simulink model "ObstacleAvoidance"  (R2023a)
settings: Solver=ode4  StartTime=0.0  StopTime=T_stop  RelTol=1e-4  AbsTol=1e-4
StartFcn:
  | close all;
  | rho_cfrp = 6.32;
  | Ts = 1e-4;
  | Tsc = Ts;
undefined symbols (not defined in the file): k_air, Kii, Kiw, Kpi, Kpw, l_bat, miu_air, Opacity, p, planedepth, planex, planey, pr_air, T_stop, Temp, Vdc, X, xrot, Y, yrot, Z, zrot
libraries: sm_lib x356, nesl_utility x78, fl_lib x65, ee_lib x17, slpidlib x8, eeBldcCurrentController x4, eePwmGenerator x4, eeGeneralControl x4, test_library x4, batteryecm_lib x1
(part 1 of 8)
settings Model: Creator=tianwang  LastModifiedBy=ashih
settings SolverCC: AlgebraicLoopSolver=TrustRegion
settings OptimizationCC: DefaultParameterBehavior=Inlined  EnhancedBackFolding=on  PassReuseOutputArgsThreshold=0  OptimizeBlockOrder=speed  DifferentSizesBufferReuse=on  OptimizationCustomize=off
settings DebuggingCC: ParameterTunabilityLossMsg=error  UnconnectedInputMsg=warning  UnconnectedOutputMsg=warning  UnconnectedLineMsg=warning
settings ModelReferenceCC: EnableRefExpFcnMdlSchedulingChecks=on
settings SFSimCC: MATLABDynamicMemAlloc=off  CustomCodeUndefinedFunction=UseInterfaceOnly
settings RTWCC: GenerateReport=on  LaunchReport=on
settings CodeAppCC: ForceParamTrailComments=on  OperatorAnnotations=on
settings SimscapeCC: SimscapeLogType=all  SimscapeLogToSDI=on
settings DiagnosticsConfigSet: SimMechanicsRigidlyBoundBlock=none
settings ExplorerConfigSet: InternalSimMechanicsExplorerSettings="<ExplorerConfiguration><canonicalview>default</canonicalview><AnimationSetting><BasePlaybackSpeed>1.0</BasePlaybackSpeed><PlaybackSpeedFactor>1.0</PlaybackSpeedFactor></AnimationSetting><TilePanel><TileInfo><Tiles Columns=\"2\" Count=\"4\" Rows=\"2\"><Column Weight=\"0.5\"/><Column Weight=\"0.5\"/><Row Weight=\"0.4994\"/><Row Weight=\"0.5006\"/><Tile Height=\"1\" Width=\"1\" X=\"0\" Y=\"0\"/><Tile Height=\"1\" Width=\"1\" X=\"0\" Y=\"1\"/><Tile Height=\"1\" Width=\"1\" X=\"1\" Y=\"0\"/><Tile Height=\"1\" Width=\"1\" X=\"1\" Y=\"1\"/></Tiles></TileInfo><SceneInfo><SceneViewer><BGColor><R>0.60000002384185791</R><G>0.60000002384185791</G><B>0.60000002384185791</B></BGColor><Camera><DoPerspective>on</DoPerspective><Position><X>8.22328992273070902</X><Y>-3.04373425990231006</Y><Z>6.27152489428823401</Z></Position><Center><X>9.05691553848198261</X><Y>-7.3270363958746092</Y><Z>5.30243470030074171</Z></Center><Up><X>-0.0530873355813747533</X><Y>-0.230177435667943048</Y><Z>0.971699584702083063</Z></Up><ViewLimDist>1</ViewLimDist><YLim>0.466307658154998583</YLim><XLim>0.890324884305486508</XLim></Camera></SceneViewer><SceneViewer><BGColor><R>0.60000002384185791</R><G>0.60000002384185791</G><B>0.60000002384185791</B></BGColor><Camera><DoPerspective>off</DoPerspective><Position><X>5.00000000638571862</X><Y>-4.9999998855435237</Y><Z>12.4219790158057197</Z></Position><Center><X>5.00000000638571862</X><Y>-4.9999998855435237</Y><Z>2.97750008320821635</Z></Center><Up><X>0</X><Y>1</Y><Z>-0</Z></Up><ViewLimDist>1</ViewLimDist><YLim>5.66500000000000004</YLim><XLim>10.7904761904761894</XLim></Camera></SceneViewer><SceneViewer><BGColor><R>0.60000002384185791</R><G>0.60000002384185791</G><B>0.60000002384185791</B></BGColor><Camera><DoPerspective>off</DoPerspective><Position><X>-3.2794800033410807</X><Y>-5.06394715817210095</Y><Z>8.07533001389897898</Z></Position><Center><X>6.09563527499397484</X><Y>-5.35335986326467594</Y><Z>2.36240522021341448</Z></Center><Up><X>0.520298147861809168</X><Y>-0.00298968077239869512</Y><Z>0.853979448898186555</Z></Up><ViewLimDist>1</ViewLimDist><YLim>6.68440638643798035</YLim><XLim>12.762589759308792</XLim></Camera></SceneViewer><SceneViewer><BGColor><R>0.60000002384185791</R><G>0.60000002384185791</G><B>0.60000002384185791</B></BGColor><Camera><DoPerspective>off</DoPerspective><Position><X>11.1167954202289536</X><Y>-11.8295490480063652</Y><Z>6.79598621935422287</Z></Position><Center><X>5.09667302982083292</X><Y>-5.80942665759825161</Y><Z>0.775863828946114831</Z></Center><Up><X>-0.408248290463863073</X><Y>0.408248290463863073</Y><Z>0.816496580927726145</Z></Up><ViewLimDist>1</ViewLimDist><YLim>6.85015205426348484</YLim><XLim>13.047908674787589</XLim></Camera></SceneViewer></SceneInfo></TilePanel><MechEditorPanel><Cameras><Camera><Id>Camera1</Id><Value><Name>ride on the drone</Name><NativeCamera><PositionKeyframeSet><Keyframe><Time>0</Time><Value><X>-0.98102517823773216</X><Y>-5.4713411967234187</Y><Z>0.96761679727529326</Z></Value></Keyframe><Keyframe><Time>0.76000000000000001</Time><Value><X>-0.99261906360083585</X><Y>-5.5052148317158611</Y><Z>1.498055339667419</Z></Value></Keyframe><Keyframe><Time>1.74</Time><Value><X>-0.98102517823773216</X><Y>-5.555286722446434</Y><Z>3.1315459048019139</Z></Value></Keyframe><Keyframe><Time>2.5800000000000001</Time><Value><X>1.7790839250037722</X><Y>-5.5473623226265607</Y><Z>4.3656146773892459</Z></Value></Keyframe><Keyframe><Time>3.2800000000000002</Time><Value><X>2.7284590777804434</X><Y>-5.6139691649844634</Y><Z>5.2937584542701197</Z></Value></Keyframe><Keyframe><Time>5.6400000000000006</Time><Value><X>4.5026745101835584</X><Y>-5.6457503851239217</Y><Z>5.4148655689845642</Z></Value></Keyframe><Keyframe><Time>7.2960000000000003</Time><Value><X>7.6384098935542299</X><Y>-4.5525145479815734</Y><Z>8.3976329181318174</Z></Value></Keyframe><Keyframe><Time>11.92</Time><Value><X>7.6384098935542299</X><Y>-4.5525145479815734</Y><Z>8.3976329181318174</Z></Value></Keyframe><Keyframe><Time>13.108000000000001</Time><Value><X>8.223289922730709</X><Y>-3.0437342599023101</Y><Z>6.271524894288234</Z></Value></Keyframe></PositionKeyframeSet><CenterKeyframeSet><Keyframe><Time>0</Time><Value><X>7.5000000000000009</X><Y>-5.4713411967234187</Y><Z>0.96761679727529326</Z></Value></Keyframe><Keyframe><Time>0.76000000000000001</Time><Value><X>7.5000000045737156</X><Y>-5.5086734535529693</Y><Z>1.3291220515700248</Z></Value></Keyframe><Keyframe><Time>1.74</Time><Value><X>7.5000000000000009</X><Y>-5.555286722446434</Y><Z>3.1315459048019139</Z></Value></Keyframe><Keyframe><Time>2.5800000000000001</Time><Value><X>7.5</X><Y>-5.5473623226265607</Y><Z>4.3656146773892459</Z></Value></Keyframe><Keyframe><Time>3.2800000000000002</Time><Value><X>7.5</X><Y>-5.6139691649844634</Y><Z>5.2937584542701197</Z></Value></Keyframe><Keyframe><Time>5.6400000000000006</Time><Value><X>7.5</X><Y>-5.6457503851239217</Y><Z>5.4148655689845642</Z></Value></Keyframe><Keyframe><Time>7.2960000000000003</Time><Value><X>7.7294479865124739</X><Y>-4.754055561900703</Y><Z>6.0049999141429025</Z></Value></Keyframe><Keyframe><Time>11.92</Time><Value><X>7.7294479865124739</X><Y>-4.754055561900703</Y><Z>6.0049999141429016</Z></Value></Keyframe><Keyframe><Time>13.108000000000001</Time><Value><X>9.0569155384819826</X><Y>-7.3270363958746092</Y><Z>5.3024347003007417</Z></Value></Keyframe></CenterKeyframeSet><UpVectorKeyframeSet><Keyframe><Time>0</Time><Value><X>0</X><Y>0</Y><Z>1</Z></Value></Keyframe><Keyframe><Time>0.76000000000000001</Time><Value><X>0.019887839858441288</X><Y>-8.0993291557236055e-06</Y><Z>0.99980221732108898</Z></Value></Keyframe><Keyframe><Time>1.74</Time><Value><X>0</X><Y>0</Y><Z>1</Z></Value></Keyframe><Keyframe><Time>2.5800000000000001</Time><Value><X>0</X><Y>0</Y><Z>1</Z></Value></Keyframe><Keyframe><Time>3.2800000000000002</Time><Value><X>0</X><Y>0</Y><Z>1</Z></Value></Keyframe><Keyframe><Time>5.6400000000000006</Time><Value><X>0</X><Y>0</Y><Z>1</Z></Value></Keyframe><Keyframe><Time>7.2960000000000003</Time><Value><X>0.99863980522167117</X><Y>-0.032540807195370107</Y><Z>0.040738621649443037</Z></Value></Keyframe><Keyframe><Time>11.92</Time><Value><X>0.99863980522167128</X><Y>-0.0325408071953701</Y><Z>0.040738621649443113</Z></Value></Keyframe><Keyframe><Time>13.108000000000001</Time><Value><X>-0.053087335581374753</X><Y>-0.23017743566794305</Y><Z>0.97169958470208306</Z></Value></Keyframe></UpVectorKeyframeSet></NativeCamera></Value></Camera></Cameras><GfxPanelCameraMap><MapElement CameraMLId=\"Camera1\" GfxPanelIndex=\"0\"/></GfxPanelCameraMap><VideoCreator><PlaybackSpeedRatio>1.0</PlaybackSpeedRatio><FrameRate>60</FrameRate><VideoFormat>MPEG-4</VideoFormat><FrameSize>[1920 1080]</FrameSize></VideoCreator></MechEditorPanel></ExplorerConfiguration>"

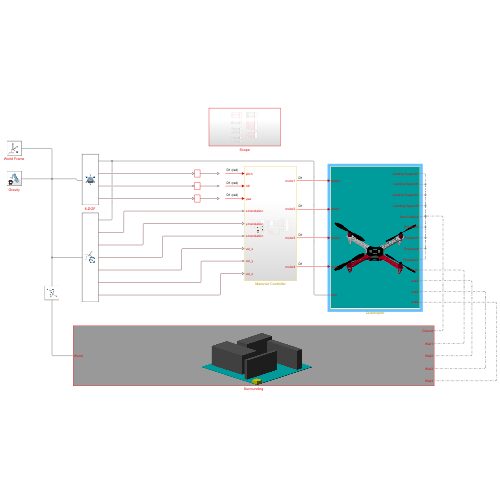
[thumbnail: Simulink's stored preview of the top-level diagram]
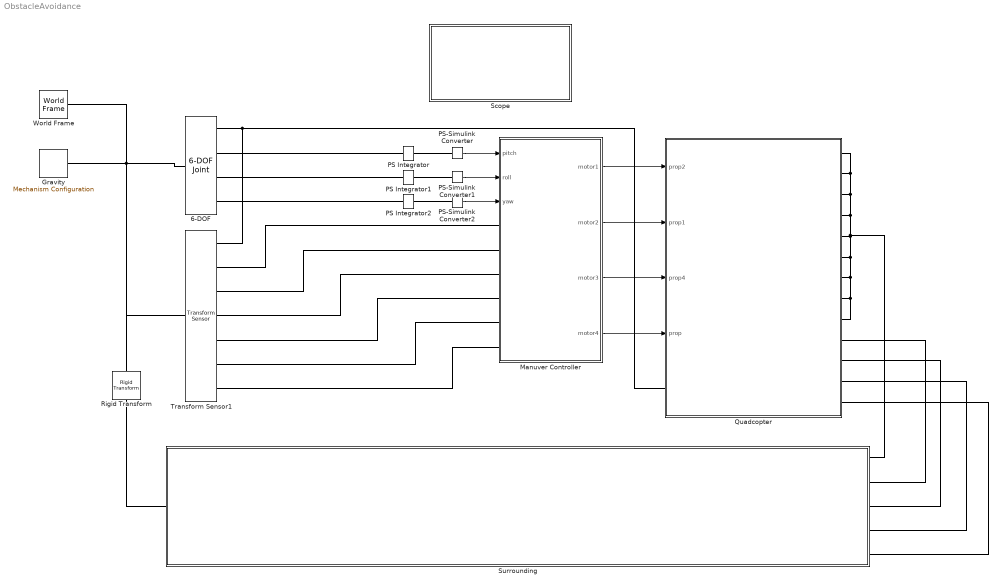
== system ObstacleAvoidance ==
  6-DOF : sm_lib/Joints/6-DOF Joint  JointMode=Normal  SenseConstraintForce=off  SenseConstraintForceX=off  SenseConstraintForceY=off  SenseConstraintForceZ=off  SenseConstraintTorque=off  SenseConstraintTorqueX=off  SenseConstraintTorqueY=off  SenseConstraintTorqueZ=off  SenseTotalForce=off  SenseTotalForceX=off  SenseTotalForceY=off  SenseTotalForceZ=off  SenseTotalTorque=off  SenseTotalTorqueX=off  SenseTotalTorqueY=off  SenseTotalTorqueZ=off  CompositeWrenchDir=FollowerOnBase  CompositeWrenchFrame=BaseFrame  PxEquilibriumPosition=0  PxEquilibriumPositionUnits=m  PxSpringStiffness=0  PxSpringStiffnessUnits=N/m  PxDampingCoefficient=0  PxDampingCoefficientUnits=N/(m/s)  PxTorqueActuationMode=NoTorque  PxMotionActuationMode=ComputedMotion  PxSensePosition=off  PxSenseVelocity=off  PxSenseAcceleration=off  PxSenseTorqueForce=off  PxSenseLowerLimitTorqueForce=off  PxSenseUpperLimitTorqueForce=off  PxLowerLimitSpecify=off  PxLowerLimitBound=-1  PxLowerLimitBoundUnits=m  PxLowerLimitStiffness=1e6  PxLowerLimitStiffnessUnits=N/m  PxLowerLimitDamping=1e3  PxLowerLimitDampingUnits=N/(m/s)  PxLowerLimitTransitionRegionWidth=1e-4  PxLowerLimitTransitionRegionWidthUnits=m  PxUpperLimitSpecify=off  PxUpperLimitBound=1  PxUpperLimitBoundUnits=m  PxUpperLimitStiffness=1e6  PxUpperLimitStiffnessUnits=N/m  PxUpperLimitDamping=1e3  PxUpperLimitDampingUnits=N/(m/s)  PxUpperLimitTransitionRegionWidth=1e-4  PxUpperLimitTransitionRegionWidthUnits=m  PxPositionTargetSpecify=on  PxPositionTargetPriority=High  PxPositionTargetValue=initial_x  PxPositionTargetValueUnits=m  PxVelocityTargetSpecify=off  PxVelocityTargetPriority=High  PxVelocityTargetValue=0  PxVelocityTargetValueUnits=m/s  PyEquilibriumPosition=0  PyEquilibriumPositionUnits=m  PySpringStiffness=0  PySpringStiffnessUnits=N/m  PyDampingCoefficient=0  PyDampingCoefficientUnits=N/(m/s)  PyTorqueActuationMode=NoTorque  PyMotionActuationMode=ComputedMotion  PySensePosition=off  PySenseVelocity=off  PySenseAcceleration=off  PySenseTorqueForce=off  PySenseLowerLimitTorqueForce=off  PySenseUpperLimitTorqueForce=off  PyLowerLimitSpecify=off  PyLowerLimitBound=-1  PyLowerLimitBoundUnits=m  PyLowerLimitStiffness=1e6  PyLowerLimitStiffnessUnits=N/m  PyLowerLimitDamping=1e3  PyLowerLimitDampingUnits=N/(m/s)  PyLowerLimitTransitionRegionWidth=1e-4  PyLowerLimitTransitionRegionWidthUnits=m  PyUpperLimitSpecify=off  PyUpperLimitBound=1  PyUpperLimitBoundUnits=m  PyUpperLimitStiffness=1e6  PyUpperLimitStiffnessUnits=N/m  PyUpperLimitDamping=1e3  PyUpperLimitDampingUnits=N/(m/s)  PyUpperLimitTransitionRegionWidth=1e-4  PyUpperLimitTransitionRegionWidthUnits=m  PyPositionTargetSpecify=on  PyPositionTargetPriority=High  PyPositionTargetValue=initial_y  PyPositionTargetValueUnits=m  PyVelocityTargetSpecify=off  PyVelocityTargetPriority=High  PyVelocityTargetValue=0  PyVelocityTargetValueUnits=m/s  PzEquilibriumPosition=0  PzEquilibriumPositionUnits=m  PzSpringStiffness=0  PzSpringStiffnessUnits=N/m  PzDampingCoefficient=0  PzDampingCoefficientUnits=N/(m/s)  PzTorqueActuationMode=NoTorque  PzMotionActuationMode=ComputedMotion  PzSensePosition=off  PzSenseVelocity=off  PzSenseAcceleration=off  PzSenseTorqueForce=off  PzSenseLowerLimitTorqueForce=off  PzSenseUpperLimitTorqueForce=off  PzLowerLimitSpecify=off  PzLowerLimitBound=-1  PzLowerLimitBoundUnits=m  PzLowerLimitStiffness=1e6  PzLowerLimitStiffnessUnits=N/m  PzLowerLimitDamping=1e3  PzLowerLimitDampingUnits=N/(m/s)  PzLowerLimitTransitionRegionWidth=1e-4  PzLowerLimitTransitionRegionWidthUnits=m  PzUpperLimitSpecify=off  PzUpperLimitBound=1  PzUpperLimitBoundUnits=m  PzUpperLimitStiffness=1e6  PzUpperLimitStiffnessUnits=N/m  PzUpperLimitDamping=1e3  PzUpperLimitDampingUnits=N/(m/s)  PzUpperLimitTransitionRegionWidth=1e-4  PzUpperLimitTransitionRegionWidthUnits=m  PzPositionTargetSpecify=on  PzPositionTargetPriority=High  PzPositionTargetValue=z0  PzPositionTargetValueUnits=m  PzVelocityTargetSpecify=off  PzVelocityTargetPriority=High  PzVelocityTargetValue=0  PzVelocityTargetValueUnits=m/s  SphEqPosRotationMethod=None  SphEqPosRotationAngleUnits=deg  SphEqPosRotationStandardAxis=+Z  SphEqPosRotationAngle=0.0  SphEqPosRotationArbitraryAxis=[0 0 1]  SphEqPosFollAlignAxisA=+X  SphEqPosBaseAlignAxisA=+Y  SphEqPosFollAlignAxisB=+Y  SphEqPosBaseAlignAxisB=+Z  SphEqPosRotationSequenceAxes=FollowerAxes  SphEqPosRotationSequence=XYX  SphEqPosRotationSequenceAngles=[0 0 0]  SphEqPosRotationSequenceAnglesUnits=deg  SphEqPosRotationMatrix=[1 0 0; 0 1 0; 0 0 1]  SphEqPosQuaternion=[1 0 0 0]  SphSpringStiffness=0  SphSpringStiffnessUnits=N*m/deg  SphDampingCoefficient=0  SphDampingCoefficientUnits=N*m/(deg/s)  SphActuateTorqueX=off  SphActuateTorqueY=off  SphActuateTorqueZ=off  SphActuateTorque=off  SphTorqueActuationMode=NoTorque  SphMotionActuationMode=ComputedMotion  SphActuationFrame=BaseFrame  SphSensePosition=off  SphSenseVelocityX=on  SphSenseVelocityY=on  SphSenseVelocityZ=on  SphSenseVelocity=off  SphSenseAccelerationX=off  SphSenseAccelerationY=off  SphSenseAccelerationZ=off  SphSenseAcceleration=off  SphSenseTorqueX=off  SphSenseTorqueY=off  SphSenseTorqueZ=off  SphSenseTorqueForce=off  SphSenseLowerLimitTorqueMag=off  SphSenseUpperLimitTorqueMag=off  SphSensingFrame=BaseFrame  SphLowerLimitSpecify=off  SphLowerLimitBound=15  SphLowerLimitBoundUnits=deg  SphLowerLimitStiffness=1e4  SphLowerLimitStiffnessUnits=N*m/deg  SphLowerLimitDamping=10  SphLowerLimitDampingUnits=N*m/(deg/s)  SphLowerLimitTransitionRegionWidth=0.1  SphLowerLimitTransitionRegionWidthUnits=deg  SphUpperLimitSpecify=off  SphUpperLimitBound=45  SphUpperLimitBoundUnits=deg  SphUpperLimitStiffness=1e4  SphUpperLimitStiffnessUnits=N*m/deg  SphUpperLimitDamping=10  SphUpperLimitDampingUnits=N*m/(deg/s)  SphUpperLimitTransitionRegionWidth=0.1  SphUpperLimitTransitionRegionWidthUnits=deg  SphPositionTargetRotationMethod=RotationSequence  SphPositionTargetRotationAngleUnits=deg  SphPositionTargetRotationStandardAxis=+Y  SphPositionTargetRotationAngle=0  SphPositionTargetRotationArbitraryAxis=[0 0 1]  SphPositionTargetFollAlignAxisA=+X  SphPositionTargetBaseAlignAxisA=+Y  SphPositionTargetFollAlignAxisB=+Y  SphPositionTargetBaseAlignAxisB=+Z  SphPositionTargetRotationSequenceAxes=FollowerAxes  SphPositionTargetRotationSequence=XYZ  SphPositionTargetRotationSequenceAngles=[xrot yrot zrot]  SphPositionTargetRotationSequenceAnglesUnits=deg  SphPositionTargetRotationMatrix=[1 0 0; 0 1 0; 0 0 1]  SphPositionTargetQuaternion=[1 0 0 0]  SphPositionTargetSpecify=on  SphPositionTargetPriority=High  SphVelocityTargetValue=[0 0 0]  SphVelocityTargetValueUnits=deg/s  SphVelocityTargetSpecify=off  SphVelocityTargetPriority=High  SphVelocityTargetInFollowerFrame=on
  Gravity : sm_lib/Utilities/Mechanism Configuration  UniformGravity=Constant  GravityVector=[0 0 -9.80665]  GravityVectorUnits=m/s^2  LinearizationDelta=0.001  JointModeTransitionNonlinearIterations=2
  Manuver Controller : Subsystem
  PS Integrator : fl_lib/Physical Signals/Linear Operators/PS Integrator  reset_method=foundation.enum.IntegratorResetSpec.None  initial_condition_spec=foundation.enum.IntegratorICSpec.Internal  saturation_spec=foundation.enum.IntegratorSaturationSpec.None  saturation_source_spec=foundation.enum.IntegratorSaturationSourceSpec.Internal  x0=0 rad  xu=inf s  xl=-inf s
  PS Integrator1 : fl_lib/Physical Signals/Linear Operators/PS Integrator  reset_method=foundation.enum.IntegratorResetSpec.None  initial_condition_spec=foundation.enum.IntegratorICSpec.Internal  saturation_spec=foundation.enum.IntegratorSaturationSpec.None  saturation_source_spec=foundation.enum.IntegratorSaturationSourceSpec.Internal  x0=0 rad  xu=inf s  xl=-inf s
  PS Integrator2 : fl_lib/Physical Signals/Linear Operators/PS Integrator  reset_method=foundation.enum.IntegratorResetSpec.None  initial_condition_spec=foundation.enum.IntegratorICSpec.Internal  saturation_spec=foundation.enum.IntegratorSaturationSpec.None  saturation_source_spec=foundation.enum.IntegratorSaturationSourceSpec.Internal  x0=0 rad  xu=inf s  xl=-inf s
  PS-Simulink Converter : nesl_utility/PS-Simulink Converter  PhysicalDomain=network_engine_domain  SubClassName=ps_output  LeftPortType=input  RightPortType=output  PseudoPeriodic=off  Frequencies=[]  VectorFormat=1-D array  Unit=inherit  AffineConversion=off
  PS-Simulink Converter1 : nesl_utility/PS-Simulink Converter  PhysicalDomain=network_engine_domain  SubClassName=ps_output  LeftPortType=input  RightPortType=output  PseudoPeriodic=off  Frequencies=[]  VectorFormat=1-D array  Unit=inherit  AffineConversion=off
  PS-Simulink Converter2 : nesl_utility/PS-Simulink Converter  PhysicalDomain=network_engine_domain  SubClassName=ps_output  LeftPortType=input  RightPortType=output  PseudoPeriodic=off  Frequencies=[]  VectorFormat=1-D array  Unit=inherit  AffineConversion=off
  Quadcopter : Subsystem
      mask Display: image('quad.PNG'); % Use "Edit Image" on toolstrip to change.
  Rigid Transform : sm_lib/Frames and Transforms/Rigid Transform  TranslationMethod=Cartesian  TranslationStandardOffset=0.05  TranslationStandardOffsetUnits=m  TranslationStandardAxis=-Z  TranslationCartesianOffset=[-5 5 -0.05]  TranslationCartesianOffsetUnits=m  TranslationROffset=0  TranslationROffsetUnits=m  TranslationZOffset=0  TranslationZOffsetUnits=m  TranslationThetaOffset=0  TranslationThetaOffsetUnits=deg  RotationMethod=None  RotationAngleUnits=deg  RotationStandardAxis=+Z  RotationAngle=0.0  RotationArbitraryAxis=[0 0 1]  FollAlignAxisA=+X  BaseAlignAxisA=+Y  FollAlignAxisB=+Y  BaseAlignAxisB=+Z  RotationSequenceAxes=FollowerAxes  RotationSequence=XYX  RotationSequenceAngles=[0 0 0]  RotationSequenceAnglesUnits=deg  RotationMatrix=[1 0 0; 0 1 0; 0 0 1]  Quaternion=[1 0 0 0]
  "Scope " : Subsystem
  Surrounding : Subsystem
      mask Display: image('surrounding.PNG'); % Use "Edit Image" on toolstrip to change.
  Transform Sensor1 : sm_lib/Frames and Transforms/Transform Sensor  MeasurementFrame=NonRotatingBase  RotationSequence=XYX  SenseAngle=off  SenseAxis=off  SenseQ=off  SenseR=off  SenseRotationSequence=off  SenseOmegaX=off  SenseOmegaY=off  SenseOmegaZ=off  SenseQDot=off  SenseRDot=off  SenseRotationSequenceDot=off  SenseAlphaX=off  SenseAlphaY=off  SenseAlphaZ=off  SenseQDDot=off  SenseRDDot=off  SenseX=on  SenseY=on  SenseZ=on  SenseRad=off  SenseAzim=off  SenseDist=off  SenseInc=off  SenseXDot=on  SenseYDot=on  SenseZDot=on  SenseRadDot=off  SenseAzimDot=off  SenseDistDot=off  SenseIncDot=off  SenseXDDot=off  SenseYDDot=off  SenseZDDot=off  SenseRadDDot=off  SenseAzimDDot=off  SenseDistDDot=off  SenseIncDDot=off
  World Frame : sm_lib/Frames and Transforms/World Frame
  wires:
  PS-Simulink Converter/1 -> Manuver Controller/1(pitch)
  PS-Simulink Converter1/1 -> Manuver Controller/2(roll)
  PS-Simulink Converter2/1 -> Manuver Controller/3(yaw)
  Manuver Controller/1(motor1) -> Quadcopter/1(prop2)
  Manuver Controller/2(motor2) -> Quadcopter/2("prop1 ")
  Manuver Controller/3(motor3) -> Quadcopter/3(prop4)
  Manuver Controller/4(motor4) -> Quadcopter/4(prop)
  connections:
  Quadcopter/LConn1 -- Transform Sensor1/RConn1 -- 6-DOF/RConn1
  Gravity/RConn1 -- Rigid Transform/RConn1 -- Transform Sensor1/LConn1 -- World Frame/RConn1 -- 6-DOF/LConn1
  Transform Sensor1/RConn2 -- Manuver Controller/LConn1
  PS Integrator/LConn1 -- 6-DOF/RConn2
  PS Integrator1/LConn1 -- 6-DOF/RConn3
  6-DOF/RConn4 -- PS Integrator2/LConn1
  PS-Simulink Converter2/LConn1 -- PS Integrator2/RConn1
  PS-Simulink Converter1/LConn1 -- PS Integrator1/RConn1
  PS-Simulink Converter/LConn1 -- PS Integrator/RConn1
  Transform Sensor1/RConn3 -- Manuver Controller/LConn2
  Transform Sensor1/RConn4 -- Manuver Controller/LConn3
  Transform Sensor1/RConn5 -- Manuver Controller/LConn4
  Transform Sensor1/RConn6 -- Manuver Controller/LConn5
  Transform Sensor1/RConn7 -- Manuver Controller/LConn6
  Quadcopter/RConn9 -- Quadcopter/RConn1 -- Quadcopter/RConn2 -- Quadcopter/RConn3 -- Quadcopter/RConn4 -- Surrounding/RConn1 -- Quadcopter/RConn5 -- Quadcopter/RConn6 -- Quadcopter/RConn7 -- Quadcopter/RConn8
  Surrounding/LConn1 -- Rigid Transform/LConn1
  Quadcopter/RConn10 -- Surrounding/RConn2
  Quadcopter/RConn11 -- Surrounding/RConn3
  Quadcopter/RConn12 -- Surrounding/RConn4
  Quadcopter/RConn13 -- Surrounding/RConn5

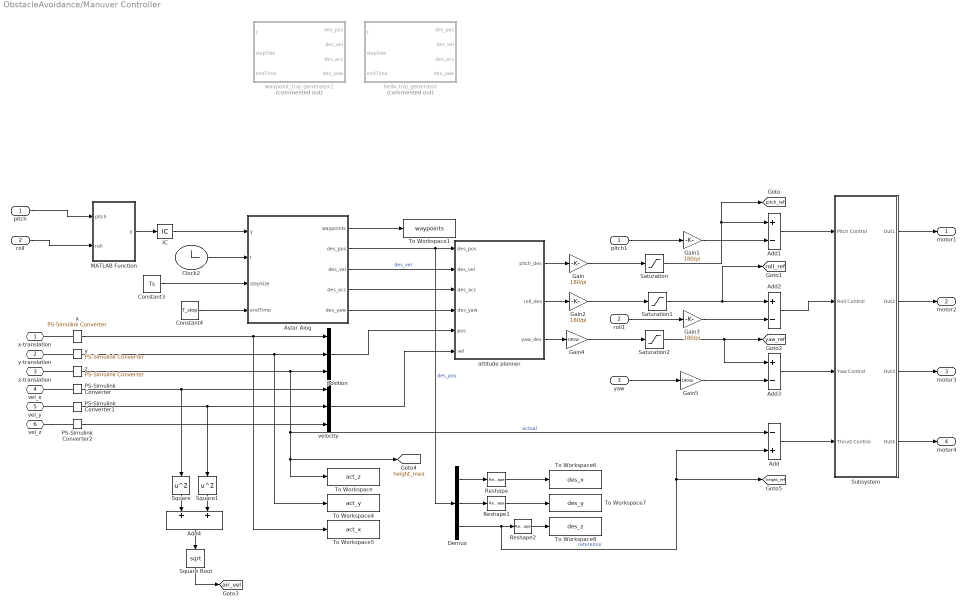
== system ObstacleAvoidance/Manuver Controller ==
  pitch : Inport
  roll : Inport  Port=2
  yaw : Inport  Port=3
  Add : Sum  Inputs=-+
  Add1 : Sum  Inputs=+-
  Add2 : Sum  Inputs=+-
  Add3 : Sum  Inputs=+-
  Add4 : Sum
  Astar Alog : MATLAB Function  TreatAsAtomicUnit=on
  Clock2 : Clock
  Constant3 : Constant  Value=Ts
  Constant4 : Constant  Value=T_stop
  Demux : Demux  Outputs=3
  Gain{,1..5} (6 alike) : Gain  Gain=180/pi
  IC : InitialCondition  Value=0
  MATLAB Function : MATLAB Function  TreatAsAtomicUnit=on
  PS-Simulink Converter : nesl_utility/PS-Simulink Converter  PhysicalDomain=network_engine_domain  SubClassName=ps_output  LeftPortType=input  RightPortType=output  PseudoPeriodic=off  Frequencies=[]  VectorFormat=1-D array  Unit=inherit  AffineConversion=off
  PS-Simulink Converter1 : nesl_utility/PS-Simulink Converter  PhysicalDomain=network_engine_domain  SubClassName=ps_output  LeftPortType=input  RightPortType=output  PseudoPeriodic=off  Frequencies=[]  VectorFormat=1-D array  Unit=inherit  AffineConversion=off
  PS-Simulink Converter2 : nesl_utility/PS-Simulink Converter  PhysicalDomain=network_engine_domain  SubClassName=ps_output  LeftPortType=input  RightPortType=output  PseudoPeriodic=off  Frequencies=[]  VectorFormat=1-D array  Unit=inherit  AffineConversion=off
  Reshape : Reshape
  Reshape1 : Reshape
  Reshape2 : Reshape
  Saturation : Saturate  UpperLimit=30  LowerLimit=-30
  Saturation1 : Saturate  UpperLimit=30  LowerLimit=-30
  Saturation2 : Saturate  UpperLimit=30  LowerLimit=-30
  Square : Math  Operator=square
  Square Root : Sqrt
  Square1 : Math  Operator=square
  Subsystem : Subsystem
  To Workspace : ToWorkspace  VariableName=act_z  SampleTime=-1
  To Workspace1 : ToWorkspace  VariableName=waypoints  SampleTime=-1
  To Workspace4 : ToWorkspace  VariableName=act_y  SampleTime=-1
  To Workspace5 : ToWorkspace  VariableName=act_x  SampleTime=-1
  To Workspace6 : ToWorkspace  VariableName=des_x  SampleTime=-1
  To Workspace7 : ToWorkspace  VariableName=des_y  SampleTime=-1
  To Workspace8 : ToWorkspace  VariableName=des_z  SampleTime=-1
  attitude planner : MATLAB Function  TreatAsAtomicUnit=on
  helix_traj_generator : MATLAB Function  Commented=on  TreatAsAtomicUnit=on
  pitch1 : InportShadow
  position : Mux  Inputs=3
  roll1 : InportShadow  Port=2
  velocity : Mux  Inputs=3
  waypoint_traj_generator2 : MATLAB Function  Commented=on  TreatAsAtomicUnit=on
  x : nesl_utility/PS-Simulink Converter  PhysicalDomain=network_engine_domain  SubClassName=ps_output  LeftPortType=input  RightPortType=output  PseudoPeriodic=off  Frequencies=[]  VectorFormat=1-D array  Unit=1  AffineConversion=off
  y : nesl_utility/PS-Simulink Converter  PhysicalDomain=network_engine_domain  SubClassName=ps_output  LeftPortType=input  RightPortType=output  PseudoPeriodic=off  Frequencies=[]  VectorFormat=1-D array  Unit=1  AffineConversion=off
  z : nesl_utility/PS-Simulink Converter  PhysicalDomain=network_engine_domain  SubClassName=ps_output  LeftPortType=input  RightPortType=output  PseudoPeriodic=off  Frequencies=[]  VectorFormat=1-D array  Unit=1  AffineConversion=off
  x-translation : PMIOPort  Side=Left
  y-translation : PMIOPort  Port=2  Side=Left
  z-translation : PMIOPort  Port=3  Side=Left
  vel_x : PMIOPort  Port=4  Side=Left
  vel_y : PMIOPort  Port=5  Side=Left
  vel_z : PMIOPort  Port=6  Side=Left
  motor1 : Outport
  motor2 : Outport  Port=2
  motor3 : Outport  Port=3
  motor4 : Outport  Port=4
  tag scope: air_vel=global, height_mea=global, height_ref=global, pitch_ref=global, roll_ref=global, yaw_ref=global
  wires:
  Subsystem/1(Out1) -> motor1/1
  Add1/1 -> Subsystem/1(Pitch Control)
  Add3/1 -> Subsystem/3(Yaw Control)
  attitude planner/3(yaw_des) -> Gain4/1
  velocity/1 -> attitude planner/6(vel)
  z/1 -> [height_mea], To Workspace/1, Add/1, position/3  "actual"
  PS-Simulink Converter1/1 -> Square1/1, velocity/2
  PS-Simulink Converter/1 -> Square/1, velocity/1
  PS-Simulink Converter2/1 -> velocity/3
  Gain5/1 -> Add3/2
  x/1 -> To Workspace5/1, position/1
  Gain2/1 -> Saturation1/1
  Gain4/1 -> Saturation2/1
  Add/1 -> Subsystem/4(Thrust Control)
  Subsystem/2(Out2) -> motor2/1
  Gain/1 -> Saturation/1
  Subsystem/4(Out4) -> motor4/1
  Astar Alog/5(des_yaw) -> attitude planner/4(des_yaw)
  attitude planner/2(roll_des) -> Gain2/1
  Add2/1 -> Subsystem/2(Roll Control)
  position/1 -> attitude planner/5(pos)
  attitude planner/1(pitch_des) -> Gain/1
  Astar Alog/4(des_acc) -> attitude planner/3(des_acc)
  Demux/2 -> Reshape1/1
  Demux/1 -> Reshape/1
  Astar Alog/3(des_vel) -> attitude planner/2(des_vel)  "des_vel"
  Demux/3 -> [height_ref], Add/2, Reshape2/1  "reference"
  Subsystem/3(Out3) -> motor3/1
  Astar Alog/2(des_pos) -> Demux/1, attitude planner/1(des_pos)  "des_pos"
  y/1 -> To Workspace4/1, position/2
  Constant4/1 -> Astar Alog/4(endTime)
  Constant3/1 -> Astar Alog/3(stepSize)
  Clock2/1 -> Astar Alog/2(t)
  Gain1/1 -> Add1/2
  Gain3/1 -> Add2/2
  Astar Alog/1(waypoints) -> To Workspace1/1
  Square/1 -> Add4/1
  Square1/1 -> Add4/2
  Add4/1 -> Square Root/1
  Square Root/1 -> [air_vel]
  Saturation/1 -> Add1/1, [pitch_ref]
  Saturation1/1 -> [roll_ref], Add2/1
  Saturation2/1 -> [yaw_ref], Add3/1
  MATLAB Function/1(y) -> IC/1
  pitch/1 -> MATLAB Function/1(pitch)
  roll/1 -> MATLAB Function/2(roll)
  roll1/1 -> Gain3/1
  pitch1/1 -> Gain1/1
  IC/1 -> Astar Alog/1(y)
  yaw/1 -> Gain5/1
  Reshape/1 -> To Workspace6/1
  Reshape1/1 -> To Workspace7/1
  Reshape2/1 -> To Workspace8/1
  connections:
  y/LConn1 -- y-translation/RConn1
  x/LConn1 -- x-translation/RConn1
  PS-Simulink Converter/LConn1 -- vel_x/RConn1
  z/LConn1 -- z-translation/RConn1
  PS-Simulink Converter1/LConn1 -- vel_y/RConn1
  vel_z/RConn1 -- PS-Simulink Converter2/LConn1

== system ObstacleAvoidance/Quadcopter ==
  prop2 : Inport
  "prop1 " : Inport  Port=2
  prop4 : Inport  Port=3
  prop : Inport  Port=4
  PS-Simulink Converter{,1..3} (4 alike) : nesl_utility/PS-Simulink Converter  PhysicalDomain=network_engine_domain  SubClassName=ps_output  LeftPortType=input  RightPortType=output  PseudoPeriodic=off  Frequencies=[]  VectorFormat=1-D array  Unit=inherit  AffineConversion=off
  Spatial Contact Force{,1..3} (4 alike) : sm_lib/Forces and Torques/Spatial Contact Force  SenseContactBaseRotation=off  SenseContactBaseTranslation=off  CoefficientOfDynamicFriction=0.1  CoefficientOfStaticFriction=0.25  NormalDamping=1e3  NormalDampingUnits=N/(m/s)  SenseContactSignal=off  NormalStiffness=1e6  NormalStiffnessUnits=N/m  FrictionalCriticalVelocity=1e-3  FrictionalCriticalVelocityUnits=m/s  ZeroCrossDetectContactStartAndEnd=off  SenseContactFollowerRotation=off  SenseContactFollowerTranslation=off  FrictionType=SmoothStickSlip  SenseFrictionalForceMagnitude=off  SenseNormalForceMagnitude=off  NormalForceType=SmoothSpringDamper  SenseNormalVelocity=off  SenseSeparationDistance=off  SenseTangentialVelocity=off  NormalTransitionRegionWidth=1e-4  NormalTransitionRegionWidthUnits=m
  battery : Subsystem
  propeller1 : Subsystem
      mask Display: image('prop2.PNG'); % Use "Edit Image" on toolstrip to change.
  propeller2 : Subsystem
      mask Display: image('prop1.PNG'); % Use "Edit Image" on toolstrip to change.
  "propeller3 " : Subsystem
      mask Display: image('prop4.PNG'); % Use "Edit Image" on toolstrip to change.
  propeller4 : Subsystem
      mask Display: image('prop3.PNG'); % Use "Edit Image" on toolstrip to change.
  quad_body : Subsystem  mask{GraphicOpacity=Opacity}
      mask prompts: GraphicOpacity "Detector Opacity:"
      mask TypeOptions GraphicOpacity: Spherical Solid/GraphicOpacity | Spherical Solid1/GraphicOpacity | Spherical Solid2/GraphicOpacity | Spherical Solid3/GraphicOpacity
      mask DialogControl DescGroupVar Prompt: QuadcopterBodyCollisionSetup
      mask DialogControl DescTextVar Prompt: The subsystem sets up the collision between the propeller, ground and wall.
      mask Display: image('quad_body.PNG'); % Use "Edit Image" on toolstrip to change.
  "Landing Support2 " : PMIOPort  Side=Right
  Landing Support1 : PMIOPort  Port=2  Side=Right
  arm : PMIOPort  Port=3  Side=Left
  "Landing Support4 " : PMIOPort  Port=4  Side=Right
  Landing Support3 : PMIOPort  Port=5  Side=Right
  Arm Collision : PMIOPort  Port=6  Side=Right
  Propeller2 : PMIOPort  Port=7  Side=Right
  Propeller1 : PMIOPort  Port=8  Side=Right
  Propeller4 : PMIOPort  Port=9  Side=Right
  "Propeller3 " : PMIOPort  Port=10  Side=Right
  wall1 : PMIOPort  Port=11  Side=Right
  wall2 : PMIOPort  Port=12  Side=Right
  wall3 : PMIOPort  Port=13  Side=Right
  wall4 : PMIOPort  Port=14  Side=Right
  tag scope: T1=global, T2=global, T3=global, T4=global
  wires:
  PS-Simulink Converter/1 -> [T2]
  PS-Simulink Converter1/1 -> [T4]
  PS-Simulink Converter2/1 -> [T1]
  PS-Simulink Converter3/1 -> [T3]
  prop2/1 -> propeller2/1(rpm)
  "prop1 "/1 -> propeller1/1(rpm)
  prop4/1 -> propeller4/1(rpm)
  prop/1 -> "propeller3 "/1(rpm)
  connections:
  quad_body/LConn2 -- arm/RConn1
  quad_body/LConn1 -- propeller2/LConn1
  quad_body/RConn1 -- propeller1/LConn1
  quad_body/LConn3 -- propeller4/LConn1
  quad_body/RConn3 -- "propeller3 "/LConn1
  Spatial Contact Force/RConn1 -- "Landing Support2 "/RConn1
  Spatial Contact Force3/RConn1 -- Landing Support1/RConn1
  Spatial Contact Force1/RConn1 -- "Landing Support4 "/RConn1
  "propeller3 "/RConn1 -- Spatial Contact Force2/LConn1
  quad_body/RConn2 -- Arm Collision/RConn1
  Propeller2/RConn1 -- propeller2/RConn2
  Propeller1/RConn1 -- propeller1/RConn2
  Propeller4/RConn1 -- propeller4/RConn2
  "Propeller3 "/RConn1 -- "propeller3 "/RConn2
  PS-Simulink Converter/LConn1 -- propeller2/LConn2
  PS-Simulink Converter1/LConn1 -- propeller4/LConn2
  PS-Simulink Converter2/LConn1 -- propeller1/LConn2
  PS-Simulink Converter3/LConn1 -- "propeller3 "/LConn2
  propeller1/LConn3 -- battery/LConn1 -- propeller2/LConn3 -- propeller4/LConn3 -- "propeller3 "/LConn3
  propeller1/LConn4 -- battery/RConn1 -- propeller2/LConn4 -- propeller4/LConn4 -- "propeller3 "/LConn4
  propeller2/RConn1 -- Spatial Contact Force/LConn1
  propeller4/RConn1 -- Spatial Contact Force1/LConn1
  propeller1/RConn1 -- Spatial Contact Force3/LConn1
  Spatial Contact Force2/RConn1 -- Landing Support3/RConn1
  propeller2/RConn3 -- wall1/RConn1 -- propeller1/RConn3 -- "propeller3 "/RConn3 -- propeller4/RConn3
  propeller2/RConn4 -- wall2/RConn1 -- "propeller3 "/RConn4 -- propeller1/RConn4 -- propeller4/RConn4
  propeller2/RConn5 -- wall3/RConn1 -- "propeller3 "/RConn5 -- propeller1/RConn5 -- propeller4/RConn5
  propeller2/RConn6 -- wall4/RConn1 -- "propeller3 "/RConn6 -- propeller1/RConn6 -- propeller4/RConn6

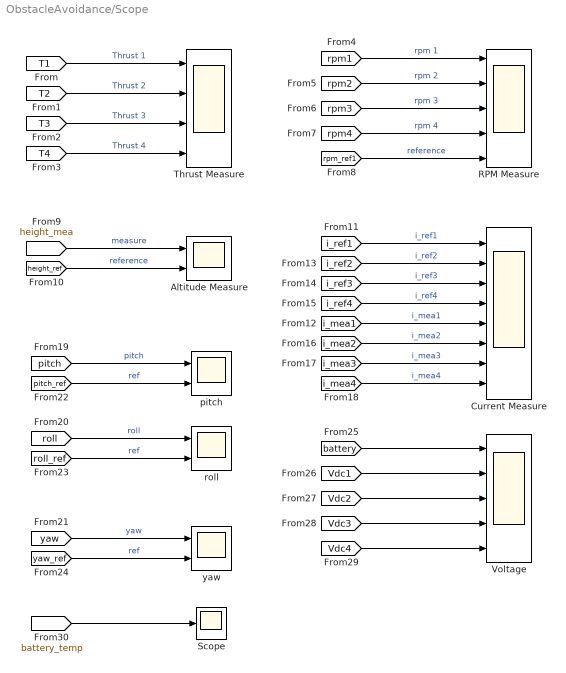
== system ObstacleAvoidance/Scope  ==
  Altitude Measure : Scope  NumInputPorts=2
  Current Measure : Scope  NumInputPorts=8
  RPM Measure : Scope  NumInputPorts=5
  Scope : Scope
  Thrust Measure : Scope  NumInputPorts=4
  Voltage : Scope  NumInputPorts=5
  pitch : Scope  NumInputPorts=2
  roll : Scope  NumInputPorts=2
  yaw : Scope  NumInputPorts=2
  wires:
  [T2] -> Thrust Measure/2  "Thrust 2"
  [T4] -> Thrust Measure/4  "Thrust 4"
  [T3] -> Thrust Measure/3  "Thrust 3"
  [T1] -> Thrust Measure/1  "Thrust 1"
  [rpm1] -> RPM Measure/1  "rpm 1"
  [rpm2] -> RPM Measure/2  "rpm 2"
  [rpm3] -> RPM Measure/3  "rpm 3"
  [rpm4] -> RPM Measure/4  "rpm 4"
  [rpm_ref1] -> RPM Measure/5  "reference"
  [height_ref] -> Altitude Measure/2  "reference"
  [height_mea] -> Altitude Measure/1  "measure"
  [i_ref1] -> Current Measure/1  "i_ref1"
  [i_ref2] -> Current Measure/2  "i_ref2"
  [i_ref3] -> Current Measure/3  "i_ref3"
  [i_ref4] -> Current Measure/4  "i_ref4"
  [i_mea1] -> Current Measure/5  "i_mea1"
  [i_mea2] -> Current Measure/6  "i_mea2"
  [i_mea3] -> Current Measure/7  "i_mea3"
  [i_mea4] -> Current Measure/8  "i_mea4"
  [pitch] -> pitch/1  "pitch"
  [roll] -> roll/1  "roll"
  [yaw] -> yaw/1  "yaw"
  [pitch_ref] -> pitch/2  "ref"
  [roll_ref] -> roll/2  "ref"
  [yaw_ref] -> yaw/2  "ref"
  [battery] -> Voltage/1
  [Vdc2] -> Voltage/3
  [Vdc1] -> Voltage/2
  [Vdc3] -> Voltage/4
  [Vdc4] -> Voltage/5
  [battery_temp] -> Scope/1

== system ObstacleAvoidance/Surrounding ==
  Destination : sm_lib/Body Elements/Brick Solid  GraphicAmbientColor=[0.15 0.15 0.15 1.0]  BasedOnType=Density  BrickDimensions=[1 1 1]  BrickDimensionsUnits=m  CenterOfMass=[0 0 0]  CenterOfMassUnits=m  GraphicDiffuseColor=[1.0 1.0 0.0]  Density=1000  DensityUnits=kg/m^3  DoExposeReferenceFrame=off  GraphicEmissiveColor=[0.0 0.0 0.0 1.0]  ExportEntireGeometry=off  SerializedFrames=<Frames><Frame><Id>Frame1</Id><Value><Name>bot</Name><Origin><Source>GeometricFeature</Source><FeatureName>-x +y -z point</FeatureName></Origin><PrimaryAxis><DefinedDirection>+Z</DefinedDirection><Source>ReferenceFrame</Source><SourceDirection>+Z</SourceDirection><FeatureName></FeatureName></PrimaryAxis><SecondaryAxis><DefinedDirection>+X</DefinedDirection><Source>ReferenceFrame</Source><SourceDirection>+X</SourceDirection><FeatureName></FeatureName></SecondaryAxis></Value></Frame></Frames>  MarkerShape=Sphere  MarkerSize=10  GraphicType=FromGeometry  InertiaType=CalculateFromGeometry  Mass=1  MassUnits=kg  MomentsOfInertia=[1 1 1]  MomentsOfInertiaUnits=kg*m^2  GraphicOpacity=1.0  ProductsOfInertia=[0 0 0]  ProductsOfInertiaUnits=kg*m^2  GraphicShininess=75  GraphicSpecularColor=[0.5 0.5 0.5 1.0]  GraphicVisPropType=SimpleVisualProperties
  Rigid Transform1 : sm_lib/Frames and Transforms/Rigid Transform  TranslationMethod=Cartesian  TranslationStandardOffset=0  TranslationStandardOffsetUnits=m  TranslationStandardAxis=+Z  TranslationCartesianOffset=[1 0 0.005]  TranslationCartesianOffsetUnits=m  TranslationROffset=0  TranslationROffsetUnits=m  TranslationZOffset=0  TranslationZOffsetUnits=m  TranslationThetaOffset=0  TranslationThetaOffsetUnits=deg  RotationMethod=None  RotationAngleUnits=deg  RotationStandardAxis=+Z  RotationAngle=0.0  RotationArbitraryAxis=[0 0 1]  FollAlignAxisA=+X  BaseAlignAxisA=+Y  FollAlignAxisB=+Y  BaseAlignAxisB=+Z  RotationSequenceAxes=FollowerAxes  RotationSequence=XYX  RotationSequenceAngles=[0 0 0]  RotationSequenceAnglesUnits=deg  RotationMatrix=[1 0 0; 0 1 0; 0 0 1]  Quaternion=[1 0 0 0]
  Rigid Transform2 : sm_lib/Frames and Transforms/Rigid Transform  TranslationMethod=Cartesian  TranslationStandardOffset=0.05  TranslationStandardOffsetUnits=m  TranslationStandardAxis=-Z  TranslationCartesianOffset=[-5 5 -0.05]  TranslationCartesianOffsetUnits=m  TranslationROffset=0  TranslationROffsetUnits=m  TranslationZOffset=0  TranslationZOffsetUnits=m  TranslationThetaOffset=0  TranslationThetaOffsetUnits=deg  RotationMethod=None  RotationAngleUnits=deg  RotationStandardAxis=+Z  RotationAngle=0.0  RotationArbitraryAxis=[0 0 1]  FollAlignAxisA=+X  BaseAlignAxisA=+Y  FollAlignAxisB=+Y  BaseAlignAxisB=+Z  RotationSequenceAxes=FollowerAxes  RotationSequence=XYX  RotationSequenceAngles=[0 0 0]  RotationSequenceAnglesUnits=deg  RotationMatrix=[1 0 0; 0 1 0; 0 0 1]  Quaternion=[1 0 0 0]
  Rigid Transform3 : sm_lib/Frames and Transforms/Rigid Transform  TranslationMethod=Cartesian  TranslationStandardOffset=0  TranslationStandardOffsetUnits=m  TranslationStandardAxis=+Z  TranslationCartesianOffset=[0 -6 0.005]  TranslationCartesianOffsetUnits=m  TranslationROffset=0  TranslationROffsetUnits=m  TranslationZOffset=0  TranslationZOffsetUnits=m  TranslationThetaOffset=0  TranslationThetaOffsetUnits=deg  RotationMethod=None  RotationAngleUnits=deg  RotationStandardAxis=+Z  RotationAngle=0.0  RotationArbitraryAxis=[0 0 1]  FollAlignAxisA=+X  BaseAlignAxisA=+Y  FollAlignAxisB=+Y  BaseAlignAxisB=+Z  RotationSequenceAxes=FollowerAxes  RotationSequence=XYX  RotationSequenceAngles=[0 0 0]  RotationSequenceAnglesUnits=deg  RotationMatrix=[1 0 0; 0 1 0; 0 0 1]  Quaternion=[1 0 0 0]
  Rigid Transform4 : sm_lib/Frames and Transforms/Rigid Transform  TranslationMethod=Cartesian  TranslationStandardOffset=0  TranslationStandardOffsetUnits=m  TranslationStandardAxis=+Z  TranslationCartesianOffset=[7.5 -4.5 0.005]  TranslationCartesianOffsetUnits=m  TranslationROffset=0  TranslationROffsetUnits=m  TranslationZOffset=0  TranslationZOffsetUnits=m  TranslationThetaOffset=0  TranslationThetaOffsetUnits=deg  RotationMethod=None  RotationAngleUnits=deg  RotationStandardAxis=+Z  RotationAngle=0.0  RotationArbitraryAxis=[0 0 1]  FollAlignAxisA=+X  BaseAlignAxisA=+Y  FollAlignAxisB=+Y  BaseAlignAxisB=+Z  RotationSequenceAxes=FollowerAxes  RotationSequence=XYX  RotationSequenceAngles=[0 0 0]  RotationSequenceAnglesUnits=deg  RotationMatrix=[1 0 0; 0 1 0; 0 0 1]  Quaternion=[1 0 0 0]
  Rigid Transform5 : sm_lib/Frames and Transforms/Rigid Transform  TranslationMethod=Cartesian  TranslationStandardOffset=0  TranslationStandardOffsetUnits=m  TranslationStandardAxis=+Z  TranslationCartesianOffset=[4 -1 0.005]  TranslationCartesianOffsetUnits=m  TranslationROffset=0  TranslationROffsetUnits=m  TranslationZOffset=0  TranslationZOffsetUnits=m  TranslationThetaOffset=0  TranslationThetaOffsetUnits=deg  RotationMethod=None  RotationAngleUnits=deg  RotationStandardAxis=+Z  RotationAngle=0.0  RotationArbitraryAxis=[0 0 1]  FollAlignAxisA=+X  BaseAlignAxisA=+Y  FollAlignAxisB=+Y  BaseAlignAxisB=+Z  RotationSequenceAxes=FollowerAxes  RotationSequence=XYX  RotationSequenceAngles=[0 0 0]  RotationSequenceAnglesUnits=deg  RotationMatrix=[1 0 0; 0 1 0; 0 0 1]  Quaternion=[1 0 0 0]
  Rigid Transform6 : sm_lib/Frames and Transforms/Rigid Transform  TranslationMethod=Cartesian  TranslationStandardOffset=0  TranslationStandardOffsetUnits=m  TranslationStandardAxis=+Z  TranslationCartesianOffset=[ 8,-9, 0.05]  TranslationCartesianOffsetUnits=m  TranslationROffset=0  TranslationROffsetUnits=m  TranslationZOffset=0  TranslationZOffsetUnits=m  TranslationThetaOffset=0  TranslationThetaOffsetUnits=deg  RotationMethod=None  RotationAngleUnits=deg  RotationStandardAxis=+Z  RotationAngle=0.0  RotationArbitraryAxis=[0 0 1]  FollAlignAxisA=+X  BaseAlignAxisA=+Y  FollAlignAxisB=+Y  BaseAlignAxisB=+Z  RotationSequenceAxes=FollowerAxes  RotationSequence=XYX  RotationSequenceAngles=[0 0 0]  RotationSequenceAnglesUnits=deg  RotationMatrix=[1 0 0; 0 1 0; 0 0 1]  Quaternion=[1 0 0 0]
  Weld Joint{,1..4} (5 alike) : sm_lib/Joints/Weld Joint  JointMode=Normal  SenseConstraintForce=off  SenseConstraintForceX=off  SenseConstraintForceY=off  SenseConstraintForceZ=off  SenseConstraintTorque=off  SenseConstraintTorqueX=off  SenseConstraintTorqueY=off  SenseConstraintTorqueZ=off  SenseTotalForce=off  SenseTotalForceX=off  SenseTotalForceY=off  SenseTotalForceZ=off  SenseTotalTorque=off  SenseTotalTorqueX=off  SenseTotalTorqueY=off  SenseTotalTorqueZ=off  CompositeWrenchDir=FollowerOnBase  CompositeWrenchFrame=BaseFrame
  ground : sm_lib/Body Elements/Brick Solid  GraphicAmbientColor=[0.15 0.15 0.15 1.0]  BasedOnType=Density  BrickDimensions=[planex planey planedepth]  BrickDimensionsUnits=m  CenterOfMass=[0 0 0]  CenterOfMassUnits=m  GraphicDiffuseColor=[0.0 0.8 0.8]  Density=1000  DensityUnits=kg/m^3  DoExposeReferenceFrame=on  GraphicEmissiveColor=[0.0 0.0 0.0 1.0]  ExportEntireGeometry=on  SerializedFrames=<Frames/>  MarkerShape=Sphere  MarkerSize=10  GraphicType=FromGeometry  InertiaType=CalculateFromGeometry  Mass=1  MassUnits=kg  MomentsOfInertia=[1 1 1]  MomentsOfInertiaUnits=kg*m^2  GraphicOpacity=1  ProductsOfInertia=[0 0 0]  ProductsOfInertiaUnits=kg*m^2  GraphicShininess=75  GraphicSpecularColor=[0.5 0.5 0.5 1.0]  GraphicVisPropType=SimpleVisualProperties
  wall1 : sm_lib/Body Elements/Brick Solid  GraphicAmbientColor=[0.15 0.15 0.15 1.0]  BasedOnType=Density  BrickDimensions=[2 5 5]  BrickDimensionsUnits=m  CenterOfMass=[0 0 0]  CenterOfMassUnits=m  GraphicDiffuseColor=[0.4 0.4 0.4]  Density=1000  DensityUnits=kg/m^3  DoExposeReferenceFrame=off  GraphicEmissiveColor=[0.0 0.0 0.0 1.0]  ExportEntireGeometry=on  SerializedFrames=<Frames><Frame><Id>Frame1</Id><Value><Name>bot</Name><Origin><Source>GeometricFeature</Source><FeatureName>-x +y -z point</FeatureName></Origin><PrimaryAxis><DefinedDirection>+Z</DefinedDirection><Source>GeometricFeature</Source><SourceDirection>+Z</SourceDirection><FeatureName>+x -y curve</FeatureName></PrimaryAxis><SecondaryAxis><DefinedDirection>+X</DefinedDirection><Source>ReferenceFrame</Source><SourceDirection>+X</SourceDirection><FeatureName></FeatureName></SecondaryAxis></Value></Frame></Frames>  MarkerShape=Sphere  MarkerSize=10  GraphicType=FromGeometry  InertiaType=CalculateFromGeometry  Mass=1  MassUnits=kg  MomentsOfInertia=[1 1 1]  MomentsOfInertiaUnits=kg*m^2  GraphicOpacity=1.0  ProductsOfInertia=[0 0 0]  ProductsOfInertiaUnits=kg*m^2  GraphicShininess=75  GraphicSpecularColor=[0.5 0.5 0.5 1.0]  GraphicVisPropType=SimpleVisualProperties
  wall2 : sm_lib/Body Elements/Brick Solid  GraphicAmbientColor=[0.15 0.15 0.15 1.0]  BasedOnType=Density  BrickDimensions=[6 3 5]  BrickDimensionsUnits=m  CenterOfMass=[0 0 0]  CenterOfMassUnits=m  GraphicDiffuseColor=[0.4 0.4 0.4]  Density=1000  DensityUnits=kg/m^3  DoExposeReferenceFrame=off  GraphicEmissiveColor=[0.0 0.0 0.0 1.0]  ExportEntireGeometry=on  SerializedFrames=<Frames><Frame><Id>Frame1</Id><Value><Name>bot</Name><Origin><Source>GeometricFeature</Source><FeatureName>-x +y -z point</FeatureName></Origin><PrimaryAxis><DefinedDirection>+Z</DefinedDirection><Source>ReferenceFrame</Source><SourceDirection>+Z</SourceDirection><FeatureName></FeatureName></PrimaryAxis><SecondaryAxis><DefinedDirection>+X</DefinedDirection><Source>ReferenceFrame</Source><SourceDirection>+X</SourceDirection><FeatureName></FeatureName></SecondaryAxis></Value></Frame></Frames>  MarkerShape=Sphere  MarkerSize=10  GraphicType=FromGeometry  InertiaType=CalculateFromGeometry  Mass=1  MassUnits=kg  MomentsOfInertia=[1 1 1]  MomentsOfInertiaUnits=kg*m^2  GraphicOpacity=1.0  ProductsOfInertia=[0 0 0]  ProductsOfInertiaUnits=kg*m^2  GraphicShininess=75  GraphicSpecularColor=[0.5 0.5 0.5 1.0]  GraphicVisPropType=SimpleVisualProperties
  wall3 : sm_lib/Body Elements/Brick Solid  GraphicAmbientColor=[0.15 0.15 0.15 1.0]  BasedOnType=Density  BrickDimensions=[0.5 5.5 5]  BrickDimensionsUnits=m  CenterOfMass=[0 0 0]  CenterOfMassUnits=m  GraphicDiffuseColor=[0.4 0.4 0.4]  Density=1000  DensityUnits=kg/m^3  DoExposeReferenceFrame=off  GraphicEmissiveColor=[0.0 0.0 0.0 1.0]  ExportEntireGeometry=on  SerializedFrames=<Frames><Frame><Id>Frame1</Id><Value><Name>bot</Name><Origin><Source>GeometricFeature</Source><FeatureName>-x +y -z point</FeatureName></Origin><PrimaryAxis><DefinedDirection>+Z</DefinedDirection><Source>ReferenceFrame</Source><SourceDirection>+Z</SourceDirection><FeatureName></FeatureName></PrimaryAxis><SecondaryAxis><DefinedDirection>+X</DefinedDirection><Source>ReferenceFrame</Source><SourceDirection>+X</SourceDirection><FeatureName></FeatureName></SecondaryAxis></Value></Frame></Frames>  MarkerShape=Sphere  MarkerSize=10  GraphicType=FromGeometry  InertiaType=CalculateFromGeometry  Mass=1  MassUnits=kg  MomentsOfInertia=[1 1 1]  MomentsOfInertiaUnits=kg*m^2  GraphicOpacity=1.0  ProductsOfInertia=[0 0 0]  ProductsOfInertiaUnits=kg*m^2  GraphicShininess=75  GraphicSpecularColor=[0.5 0.5 0.5 1.0]  GraphicVisPropType=SimpleVisualProperties
  wall4 : sm_lib/Body Elements/Brick Solid  GraphicAmbientColor=[0.15 0.15 0.15 1.0]  BasedOnType=Density  BrickDimensions=[6 1 5]  BrickDimensionsUnits=m  CenterOfMass=[0 0 0]  CenterOfMassUnits=m  GraphicDiffuseColor=[0.4 0.4 0.4]  Density=1000  DensityUnits=kg/m^3  DoExposeReferenceFrame=off  GraphicEmissiveColor=[0.0 0.0 0.0 1.0]  ExportEntireGeometry=on  SerializedFrames=<Frames><Frame><Id>Frame1</Id><Value><Name>bot</Name><Origin><Source>GeometricFeature</Source><FeatureName>-x +y -z point</FeatureName></Origin><PrimaryAxis><DefinedDirection>+Z</DefinedDirection><Source>ReferenceFrame</Source><SourceDirection>+Z</SourceDirection><FeatureName></FeatureName></PrimaryAxis><SecondaryAxis><DefinedDirection>+X</DefinedDirection><Source>ReferenceFrame</Source><SourceDirection>+X</SourceDirection><FeatureName></FeatureName></SecondaryAxis></Value></Frame></Frames>  MarkerShape=Sphere  MarkerSize=10  GraphicType=FromGeometry  InertiaType=CalculateFromGeometry  Mass=1  MassUnits=kg  MomentsOfInertia=[1 1 1]  MomentsOfInertiaUnits=kg*m^2  GraphicOpacity=1.0  ProductsOfInertia=[0 0 0]  ProductsOfInertiaUnits=kg*m^2  GraphicShininess=75  GraphicSpecularColor=[0.5 0.5 0.5 1.0]  GraphicVisPropType=SimpleVisualProperties
  World : PMIOPort  Side=Left
  Ground : PMIOPort  Port=2  Side=Right
  Wall1 : PMIOPort  Port=3  Side=Right
  Wall2 : PMIOPort  Port=4  Side=Right
  Wall3 : PMIOPort  Port=5  Side=Right
  Wall4 : PMIOPort  Port=6  Side=Right
  connections:
  Rigid Transform5/RConn1 -- wall4/LConn1
  Weld Joint2/RConn1 -- Rigid Transform4/LConn1
  Rigid Transform2/RConn1 -- Weld Joint3/LConn1 -- Weld Joint4/LConn1 -- Weld Joint2/LConn1 -- Weld Joint1/LConn1 -- Weld Joint/LConn1
  Weld Joint1/RConn1 -- Rigid Transform3/LConn1
  Rigid Transform4/RConn1 -- wall3/LConn1
  Wall4/RConn1 -- wall4/RConn1
  Wall2/RConn1 -- wall2/RConn1
  ground/RConn1 -- World/RConn1 -- Rigid Transform2/LConn1
  Rigid Transform3/RConn1 -- wall2/LConn1
  wall1/LConn1 -- Rigid Transform1/RConn1
  Rigid Transform6/RConn1 -- Destination/LConn1
  Rigid Transform1/LConn1 -- Weld Joint/RConn1
  Wall3/RConn1 -- wall3/RConn1
  Weld Joint3/RConn1 -- Rigid Transform5/LConn1
  Weld Joint4/RConn1 -- Rigid Transform6/LConn1
  ground/LConn1 -- Ground/RConn1
  Wall1/RConn1 -- wall1/RConn1
